simulink model "EsamblajeCohete2_0"  (R2023a)
settings: Solver=VariableStepAuto  StartTime=0.0  StopTime=120  RelTol=1e-3
model workspace: external: MATLAB File C:\Users\SEBASTIANDIAZPABON\OneDrive - Universidad Santo Tomás Bucaramanga\USTA\Semillero Cohete\Cohete Matlab 2.0\EsamblajeCohete2_0_DataFile.m (data not in the file)
undefined symbols (not defined in the file): smiData, X, Y, Z
libraries: sm_lib x354, nesl_utility x13, simulink x7, fuzblock x6
(part 7 of 7)

== system EsamblajeCohete2_0/Cohete/Assembly_4_RIGID/Magnet_8_RIGID ==
  ReferenceFrame : sm_lib/Frames and Transforms/Reference Frame
  Solid : sm_lib/Body Elements/File Solid  ExtGeomFileName=Magnet_Default_sldprt.STEP  UnitType=FromFile  ExtGeomFileUnits=m  StepReaderType=HEX  ExportConvexHullGeometry=off  InertiaType=Custom  Mass=smiData.Solid(5).mass  MassUnits=kg  CenterOfMass=smiData.Solid(5).CoM  CenterOfMassUnits=mm  MomentsOfInertia=smiData.Solid(5).MoI  MomentsOfInertiaUnits=kg*mm^2  ProductsOfInertia=smiData.Solid(5).PoI  ProductsOfInertiaUnits=kg*mm^2  BasedOnType=DensityFromFile  Density=1000  DensityUnits=kg/m^3  DoExposeReferenceFrame=on  SerializedFrames=<Frames/>  GraphicType=FromGeometry  MarkerShape=Sphere  MarkerSize=10  GraphicVisPropType=SimpleVisualProperties  GraphicDiffuseColor=smiData.Solid(5).color  GraphicSpecularColor=[0.5 0.5 0.5 1.0]  GraphicAmbientColor=[0.15 0.15 0.15 1.0]  GraphicEmissiveColor=[0.0 0.0 0.0 1.0]  GraphicShininess=75  GraphicOpacity=smiData.Solid(5).opacity
  F : PMIOPort  Side=Left
  connections:
  Solid/RConn1 -- ReferenceFrame/RConn1 -- F/RConn1

== system EsamblajeCohete2_0/Cohete/Assembly_4_RIGID/Magnet_9_RIGID ==
  ReferenceFrame : sm_lib/Frames and Transforms/Reference Frame
  Solid : sm_lib/Body Elements/File Solid  ExtGeomFileName=Magnet_Default_sldprt.STEP  UnitType=FromFile  ExtGeomFileUnits=m  StepReaderType=HEX  ExportConvexHullGeometry=off  InertiaType=Custom  Mass=smiData.Solid(5).mass  MassUnits=kg  CenterOfMass=smiData.Solid(5).CoM  CenterOfMassUnits=mm  MomentsOfInertia=smiData.Solid(5).MoI  MomentsOfInertiaUnits=kg*mm^2  ProductsOfInertia=smiData.Solid(5).PoI  ProductsOfInertiaUnits=kg*mm^2  BasedOnType=DensityFromFile  Density=1000  DensityUnits=kg/m^3  DoExposeReferenceFrame=on  SerializedFrames=<Frames/>  GraphicType=FromGeometry  MarkerShape=Sphere  MarkerSize=10  GraphicVisPropType=SimpleVisualProperties  GraphicDiffuseColor=smiData.Solid(5).color  GraphicSpecularColor=[0.5 0.5 0.5 1.0]  GraphicAmbientColor=[0.15 0.15 0.15 1.0]  GraphicEmissiveColor=[0.0 0.0 0.0 1.0]  GraphicShininess=75  GraphicOpacity=smiData.Solid(5).opacity
  F : PMIOPort  Side=Left
  connections:
  Solid/RConn1 -- ReferenceFrame/RConn1 -- F/RConn1

== system EsamblajeCohete2_0/Cohete/Assembly_4_RIGID/Motor_Casing_1_RIGID ==
  ReferenceFrame : sm_lib/Frames and Transforms/Reference Frame
  Solid : sm_lib/Body Elements/File Solid  ExtGeomFileName=Motor Casing_Default_sldprt.STEP  UnitType=FromFile  ExtGeomFileUnits=m  StepReaderType=HEX  ExportConvexHullGeometry=off  InertiaType=Custom  Mass=smiData.Solid(8).mass  MassUnits=kg  CenterOfMass=smiData.Solid(8).CoM  CenterOfMassUnits=mm  MomentsOfInertia=smiData.Solid(8).MoI  MomentsOfInertiaUnits=kg*mm^2  ProductsOfInertia=smiData.Solid(8).PoI  ProductsOfInertiaUnits=kg*mm^2  BasedOnType=DensityFromFile  Density=1000  DensityUnits=kg/m^3  DoExposeReferenceFrame=on  SerializedFrames=<Frames/>  GraphicType=FromGeometry  MarkerShape=Sphere  MarkerSize=10  GraphicVisPropType=SimpleVisualProperties  GraphicDiffuseColor=smiData.Solid(8).color  GraphicSpecularColor=[0.5 0.5 0.5 1.0]  GraphicAmbientColor=[0.15 0.15 0.15 1.0]  GraphicEmissiveColor=[0.0 0.0 0.0 1.0]  GraphicShininess=75  GraphicOpacity=smiData.Solid(8).opacity
  F : PMIOPort  Side=Left
  connections:
  Solid/RConn1 -- ReferenceFrame/RConn1 -- F/RConn1

== system EsamblajeCohete2_0/Cohete/Assembly_4_RIGID/Nut_2_RIGID ==
  ReferenceFrame : sm_lib/Frames and Transforms/Reference Frame
  Solid : sm_lib/Body Elements/File Solid  ExtGeomFileName=Nut_Default_sldprt.STEP  UnitType=FromFile  ExtGeomFileUnits=m  StepReaderType=HEX  ExportConvexHullGeometry=off  InertiaType=Custom  Mass=smiData.Solid(13).mass  MassUnits=kg  CenterOfMass=smiData.Solid(13).CoM  CenterOfMassUnits=mm  MomentsOfInertia=smiData.Solid(13).MoI  MomentsOfInertiaUnits=kg*mm^2  ProductsOfInertia=smiData.Solid(13).PoI  ProductsOfInertiaUnits=kg*mm^2  BasedOnType=DensityFromFile  Density=1000  DensityUnits=kg/m^3  DoExposeReferenceFrame=on  SerializedFrames=<Frames/>  GraphicType=FromGeometry  MarkerShape=Sphere  MarkerSize=10  GraphicVisPropType=SimpleVisualProperties  GraphicDiffuseColor=smiData.Solid(13).color  GraphicSpecularColor=[0.5 0.5 0.5 1.0]  GraphicAmbientColor=[0.15 0.15 0.15 1.0]  GraphicEmissiveColor=[0.0 0.0 0.0 1.0]  GraphicShininess=75  GraphicOpacity=smiData.Solid(13).opacity
  F : PMIOPort  Side=Left
  connections:
  Solid/RConn1 -- ReferenceFrame/RConn1 -- F/RConn1

== system EsamblajeCohete2_0/Cohete/Assembly_4_RIGID/Rotor_1_RIGID ==
  ReferenceFrame : sm_lib/Frames and Transforms/Reference Frame
  Solid : sm_lib/Body Elements/File Solid  ExtGeomFileName=Rotor_Default_sldprt.STEP  UnitType=FromFile  ExtGeomFileUnits=m  StepReaderType=HEX  ExportConvexHullGeometry=off  InertiaType=Custom  Mass=smiData.Solid(9).mass  MassUnits=kg  CenterOfMass=smiData.Solid(9).CoM  CenterOfMassUnits=mm  MomentsOfInertia=smiData.Solid(9).MoI  MomentsOfInertiaUnits=kg*mm^2  ProductsOfInertia=smiData.Solid(9).PoI  ProductsOfInertiaUnits=kg*mm^2  BasedOnType=DensityFromFile  Density=1000  DensityUnits=kg/m^3  DoExposeReferenceFrame=on  SerializedFrames=<Frames/>  GraphicType=FromGeometry  MarkerShape=Sphere  MarkerSize=10  GraphicVisPropType=SimpleVisualProperties  GraphicDiffuseColor=smiData.Solid(9).color  GraphicSpecularColor=[0.5 0.5 0.5 1.0]  GraphicAmbientColor=[0.15 0.15 0.15 1.0]  GraphicEmissiveColor=[0.0 0.0 0.0 1.0]  GraphicShininess=75  GraphicOpacity=smiData.Solid(9).opacity
  F : PMIOPort  Side=Left
  connections:
  Solid/RConn1 -- ReferenceFrame/RConn1 -- F/RConn1

== system EsamblajeCohete2_0/Cohete/Assembly_4_RIGID/Rotor_Cover_1_RIGID ==
  ReferenceFrame : sm_lib/Frames and Transforms/Reference Frame
  Solid : sm_lib/Body Elements/File Solid  ExtGeomFileName=Rotor Cover_Default_sldprt.STEP  UnitType=FromFile  ExtGeomFileUnits=m  StepReaderType=HEX  ExportConvexHullGeometry=off  InertiaType=Custom  Mass=smiData.Solid(11).mass  MassUnits=kg  CenterOfMass=smiData.Solid(11).CoM  CenterOfMassUnits=mm  MomentsOfInertia=smiData.Solid(11).MoI  MomentsOfInertiaUnits=kg*mm^2  ProductsOfInertia=smiData.Solid(11).PoI  ProductsOfInertiaUnits=kg*mm^2  BasedOnType=DensityFromFile  Density=1000  DensityUnits=kg/m^3  DoExposeReferenceFrame=on  SerializedFrames=<Frames/>  GraphicType=FromGeometry  MarkerShape=Sphere  MarkerSize=10  GraphicVisPropType=SimpleVisualProperties  GraphicDiffuseColor=smiData.Solid(11).color  GraphicSpecularColor=[0.5 0.5 0.5 1.0]  GraphicAmbientColor=[0.15 0.15 0.15 1.0]  GraphicEmissiveColor=[0.0 0.0 0.0 1.0]  GraphicShininess=75  GraphicOpacity=smiData.Solid(11).opacity
  F : PMIOPort  Side=Left
  connections:
  Solid/RConn1 -- ReferenceFrame/RConn1 -- F/RConn1

== system EsamblajeCohete2_0/Cohete/Assembly_4_RIGID/Stopper_Screw_1_RIGID ==
  ReferenceFrame : sm_lib/Frames and Transforms/Reference Frame
  Solid : sm_lib/Body Elements/File Solid  ExtGeomFileName=Stopper Screw_Default_sldprt.STEP  UnitType=FromFile  ExtGeomFileUnits=m  StepReaderType=HEX  ExportConvexHullGeometry=off  InertiaType=Custom  Mass=smiData.Solid(12).mass  MassUnits=kg  CenterOfMass=smiData.Solid(12).CoM  CenterOfMassUnits=mm  MomentsOfInertia=smiData.Solid(12).MoI  MomentsOfInertiaUnits=kg*mm^2  ProductsOfInertia=smiData.Solid(12).PoI  ProductsOfInertiaUnits=kg*mm^2  BasedOnType=DensityFromFile  Density=1000  DensityUnits=kg/m^3  DoExposeReferenceFrame=on  SerializedFrames=<Frames/>  GraphicType=FromGeometry  MarkerShape=Sphere  MarkerSize=10  GraphicVisPropType=SimpleVisualProperties  GraphicDiffuseColor=smiData.Solid(12).color  GraphicSpecularColor=[0.5 0.5 0.5 1.0]  GraphicAmbientColor=[0.15 0.15 0.15 1.0]  GraphicEmissiveColor=[0.0 0.0 0.0 1.0]  GraphicShininess=75  GraphicOpacity=smiData.Solid(12).opacity
  F : PMIOPort  Side=Left
  connections:
  Solid/RConn1 -- ReferenceFrame/RConn1 -- F/RConn1

== system EsamblajeCohete2_0/Cohete/Assembly_4_RIGID/e_ring_external_retaining_ring_wti_4_RIGID ==
  ReferenceFrame : sm_lib/Frames and Transforms/Reference Frame
  Solid : sm_lib/Body Elements/File Solid  ExtGeomFileName=e-ring external retaining ring_wti_Truarc X5133-14 - S0.14_sldprt.STEP  UnitType=FromFile  ExtGeomFileUnits=m  StepReaderType=HEX  ExportConvexHullGeometry=off  InertiaType=Custom  Mass=smiData.Solid(10).mass  MassUnits=kg  CenterOfMass=smiData.Solid(10).CoM  CenterOfMassUnits=in  MomentsOfInertia=smiData.Solid(10).MoI  MomentsOfInertiaUnits=kg*in^2  ProductsOfInertia=smiData.Solid(10).PoI  ProductsOfInertiaUnits=kg*in^2  BasedOnType=DensityFromFile  Density=1000  DensityUnits=kg/m^3  DoExposeReferenceFrame=on  SerializedFrames=<Frames/>  GraphicType=FromGeometry  MarkerShape=Sphere  MarkerSize=10  GraphicVisPropType=SimpleVisualProperties  GraphicDiffuseColor=smiData.Solid(10).color  GraphicSpecularColor=[0.5 0.5 0.5 1.0]  GraphicAmbientColor=[0.15 0.15 0.15 1.0]  GraphicEmissiveColor=[0.0 0.0 0.0 1.0]  GraphicShininess=75  GraphicOpacity=smiData.Solid(10).opacity
  F : PMIOPort  Side=Left
  connections:
  Solid/RConn1 -- ReferenceFrame/RConn1 -- F/RConn1

== system EsamblajeCohete2_0/Cohete/Assembly_4_RIGID/instrument_ball_bearing_68_iso_1_RIGID ==
  ReferenceFrame : sm_lib/Frames and Transforms/Reference Frame
  Solid : sm_lib/Body Elements/File Solid  ExtGeomFileName=instrument ball bearing_68_iso_ISO 1224 - 390308 - R-8-DE-NC-8_68_sldprt.STEP  UnitType=FromFile  ExtGeomFileUnits=m  StepReaderType=HEX  ExportConvexHullGeometry=off  InertiaType=Custom  Mass=smiData.Solid(14).mass  MassUnits=kg  CenterOfMass=smiData.Solid(14).CoM  CenterOfMassUnits=mm  MomentsOfInertia=smiData.Solid(14).MoI  MomentsOfInertiaUnits=kg*mm^2  ProductsOfInertia=smiData.Solid(14).PoI  ProductsOfInertiaUnits=kg*mm^2  BasedOnType=DensityFromFile  Density=1000  DensityUnits=kg/m^3  DoExposeReferenceFrame=on  SerializedFrames=<Frames/>  GraphicType=FromGeometry  MarkerShape=Sphere  MarkerSize=10  GraphicVisPropType=SimpleVisualProperties  GraphicDiffuseColor=smiData.Solid(14).color  GraphicSpecularColor=[0.5 0.5 0.5 1.0]  GraphicAmbientColor=[0.15 0.15 0.15 1.0]  GraphicEmissiveColor=[0.0 0.0 0.0 1.0]  GraphicShininess=75  GraphicOpacity=smiData.Solid(14).opacity
  F : PMIOPort  Side=Left
  connections:
  Solid/RConn1 -- ReferenceFrame/RConn1 -- F/RConn1

== system EsamblajeCohete2_0/Controlador + Planta/PID ADTITUDE/PID ATITUDE ==
  Z : Inport
  Z_error : Inport  Port=2
  Add : Sum  Inputs=+++
  Derivative : Derivative
  Integrator : Integrator
  Kda : Gain  Gain=1.5789
  Kia : Gain  Gain=0.021147
  Kpa : Gain  Gain=0.36
  Sum : Sum  Inputs=|+-
  Transfer Fcn : TransferFcn  Denominator=[1.6 0 0]
  z : Outport
  wires:
  Derivative/1 -> Add/3
  Integrator/1 -> Add/2
  Kpa/1 -> Add/1
  Sum/1 -> Kda/1, Kia/1, Kpa/1
  Z/1 -> Sum/1
  Z_error/1 -> Sum/2
  Kia/1 -> Integrator/1
  Kda/1 -> Derivative/1
  Add/1 -> Transfer Fcn/1
  Transfer Fcn/1 -> z/1

== system EsamblajeCohete2_0/Controlador + Planta/PID ADTITUDE/PID ATITUDE X ==
  X_d : Inport
  X_er : Inport  Port=2
  Add : Sum  Inputs=+++
  Add1 : Sum  Commented=on  Inputs=+-+-
  Derivative : Derivative
  Integrator : Integrator
  Kda : Gain  Gain=1.5789
  Kia : Gain  Gain=0.021147
  Kpa : Gain  Gain=0.36
  Ramp : simulink/Sources/Ramp  Commented=on  slope=0.1  start=18  InitialOutput=0
  Ramp1 : simulink/Sources/Ramp  Commented=on  slope=0.1  start=23  InitialOutput=0
  Step1 : Step  Commented=on  Time=24  After=0.12  SampleTime=0
  Step2 : Step  Commented=on  Time=24  After=0.62  SampleTime=0
  Sum : Sum  Inputs=|+-
  Sum1 : Sum  Inputs=|++
  Transfer Fcn : TransferFcn  Denominator=[1.6 0 0]
  z : Outport
  wires:
  Derivative/1 -> Add/3
  Integrator/1 -> Add/2
  Kpa/1 -> Add/1
  Sum/1 -> Kda/1, Kia/1, Kpa/1
  X_d/1 -> Sum/1
  X_er/1 -> Sum/2
  Kia/1 -> Integrator/1
  Kda/1 -> Derivative/1
  Add/1 -> Transfer Fcn/1
  Transfer Fcn/1 -> Sum1/1
  Sum1/1 -> z/1
  Ramp/1 -> Add1/1
  Ramp1/1 -> Add1/2
  Step1/1 -> Add1/3
  Step2/1 -> Add1/4
  Add1/1 -> Sum1/2

== system EsamblajeCohete2_0/Controlador + Planta/PID ADTITUDE/PID ATITUDE y  ==
  Z : Inport
  Z_error : Inport  Port=2
  Add : Sum  Inputs=+++
  Derivative : Derivative
  Integrator : Integrator
  Kda : Gain  Gain=1.5789
  Kia : Gain  Gain=0.021147
  Kpa : Gain  Gain=0.36
  Sum : Sum  Inputs=|+-
  Transfer Fcn : TransferFcn  Denominator=[1.6 0 0]
  z : Outport
  wires:
  Derivative/1 -> Add/3
  Integrator/1 -> Add/2
  Kpa/1 -> Add/1
  Sum/1 -> Kda/1, Kia/1, Kpa/1
  Z/1 -> Sum/1
  Z_error/1 -> Sum/2
  Kia/1 -> Integrator/1
  Kda/1 -> Derivative/1
  Add/1 -> Transfer Fcn/1
  Transfer Fcn/1 -> z/1

== system EsamblajeCohete2_0/Controlador + Planta/Rotation PID/PID θ ==
  θ : Inport
  θ_error : Inport  Port=2
  Add : Sum  Inputs=+++
  Derivative : Derivative
  Integrator : Integrator
  Kda : Gain  Gain=0.03947
  Kia : Gain  Gain=0.0005287
  Kpa : Gain  Gain=0.009136
  Sum : Sum  Inputs=|+-
  Transfer Fcn : TransferFcn  Denominator=[0.02 0 0]
  theta : Outport
  wires:
  Derivative/1 -> Add/3
  Integrator/1 -> Add/2
  Kpa/1 -> Add/1
  Sum/1 -> Kda/1, Kia/1, Kpa/1
  θ/1 -> Sum/1
  θ_error/1 -> Sum/2
  Kia/1 -> Integrator/1
  Kda/1 -> Derivative/1
  Add/1 -> Transfer Fcn/1
  Transfer Fcn/1 -> theta/1

== system EsamblajeCohete2_0/Controlador + Planta/Rotation PID/PID φ ==
  φ : Inport
  φ_error : Inport  Port=2
  Add : Sum  Inputs=+++
  Derivative : Derivative
  Integrator : Integrator
  Kda : Gain  Gain=0.01973
  Kia : Gain  Gain=0.00026434
  Kpa : Gain  Gain=0.0045681
  Sum : Sum  Inputs=|+-
  Transfer Fcn : TransferFcn  Denominator=[0.04 0 0]
  Out1 : Outport
  wires:
  Derivative/1 -> Add/3
  Integrator/1 -> Add/2
  Kpa/1 -> Add/1
  Sum/1 -> Kda/1, Kia/1, Kpa/1
  φ/1 -> Sum/1
  φ_error/1 -> Sum/2
  Kia/1 -> Integrator/1
  Kda/1 -> Derivative/1
  Add/1 -> Transfer Fcn/1
  Transfer Fcn/1 -> Out1/1

== system EsamblajeCohete2_0/Controlador + Planta/Rotation PID/PID ψ ==
  ψ : Inport
  ψ_error : Inport  Port=2
  Add : Sum  Inputs=+++
  Derivative : Derivative
  Integrator : Integrator
  Kda : Gain  Gain=0.03947
  Kia : Gain  Gain=0.0005287
  Kpa : Gain  Gain=0.009136
  Sum : Sum  Inputs=|+-
  Transfer Fcn : TransferFcn  Denominator=[0.02 0 0]
  theta : Outport
  wires:
  Derivative/1 -> Add/3
  Integrator/1 -> Add/2
  Kpa/1 -> Add/1
  Sum/1 -> Kda/1, Kia/1, Kpa/1
  ψ/1 -> Sum/1
  ψ_error/1 -> Sum/2
  Kia/1 -> Integrator/1
  Kda/1 -> Derivative/1
  Add/1 -> Transfer Fcn/1
  Transfer Fcn/1 -> theta/1

== system EsamblajeCohete2_0/Qudrotor Dinamics/Rotacional/θ'' ==
  Iyy : Inport
  Izz : Inport  Port=2
  Ixx : Inport  Port=3
  φ' : Inport  Port=4
  ψ' : Inport  Port=5
  L : Inport  Port=6
  U3 : Inport  Port=7
  Add : Sum  Inputs=+-
  Add1 : Sum
  Divide : Product  Inputs=*/
  Divide1 : Product  Inputs=*/
  Product : Product
  Product1 : Product  Inputs=3
  θ'' : Outport
  wires:
  Add/1 -> Divide/1
  Divide/1 -> Product1/1
  Product/1 -> Divide1/1
  Product1/1 -> Add1/1
  Divide1/1 -> Add1/2
  Add1/1 -> θ''/1
  Iyy/1 -> Divide1/2, Divide/2
  Izz/1 -> Add/1
  Ixx/1 -> Add/2
  φ'/1 -> Product1/2
  ψ'/1 -> Product1/3
  L/1 -> Product/1
  U3/1 -> Product/2

== system EsamblajeCohete2_0/Qudrotor Dinamics/Rotacional/φ'' ==
  Iyy : Inport
  Izz : Inport  Port=2
  Ixx : Inport  Port=3
  θ' : Inport  Port=4
  ψ' : Inport  Port=5
  L : Inport  Port=6
  U2 : Inport  Port=7
  Add : Sum  Inputs=+-
  Add1 : Sum
  Divide : Product  Inputs=*/
  Divide1 : Product  Inputs=*/
  Product : Product
  Product1 : Product  Inputs=3
  φ'' : Outport
  wires:
  Iyy/1 -> Add/1
  Izz/1 -> Add/2
  Add/1 -> Divide/1
  Ixx/1 -> Divide1/2, Divide/2
  Divide/1 -> Product1/1
  θ'/1 -> Product1/2
  ψ'/1 -> Product1/3
  L/1 -> Product/1
  U2/1 -> Product/2
  Product/1 -> Divide1/1
  Product1/1 -> Add1/1
  Divide1/1 -> Add1/2
  Add1/1 -> φ''/1

== system EsamblajeCohete2_0/Qudrotor Dinamics/Rotacional/ψ'' ==
  Iyy : Inport
  Izz : Inport  Port=2
  Ixx : Inport  Port=3
  φ' : Inport  Port=4
  θ' : Inport  Port=5
  L : Inport  Port=6
  U4 : Inport  Port=7
  Add : Sum  Inputs=+-
  Add1 : Sum
  Divide : Product  Inputs=*/
  Divide1 : Product  Inputs=*/
  Product : Product
  Product1 : Product  Inputs=3
  ψ'' : Outport
  wires:
  Add/1 -> Divide/1
  Divide/1 -> Product1/1
  Product/1 -> Divide1/1
  Product1/1 -> Add1/1
  Divide1/1 -> Add1/2
  Add1/1 -> ψ''/1
  Iyy/1 -> Add/2
  Ixx/1 -> Add/1
  Izz/1 -> Divide1/2, Divide/2
  φ'/1 -> Product1/2
  θ'/1 -> Product1/3
  L/1 -> Product/1
  U4/1 -> Product/2

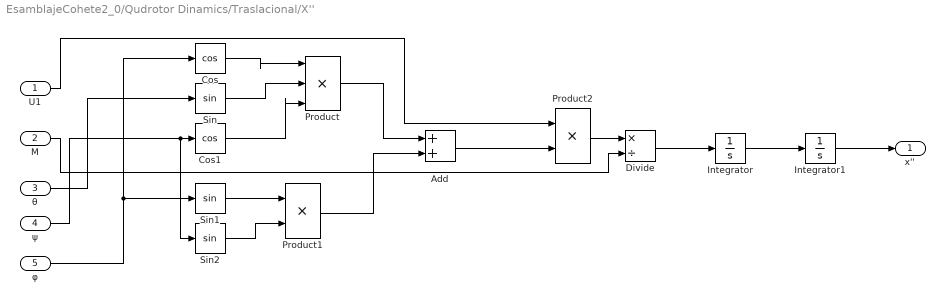
== system EsamblajeCohete2_0/Qudrotor Dinamics/Traslacional/X'' ==
  U1 : Inport
  M : Inport  Port=2
  θ : Inport  Port=3
  ψ : Inport  Port=4
  φ : Inport  Port=5
  Add : Sum
  Cos : Trigonometry  Operator=cos
  Cos1 : Trigonometry  Operator=cos
  Divide : Product  Inputs=*/
  Integrator : Integrator
  Integrator1 : Integrator
  Product : Product  Inputs=3
  Product1 : Product
  Product2 : Product
  Sin : Trigonometry
  Sin1 : Trigonometry
  Sin2 : Trigonometry
  x'' : Outport
  wires:
  φ/1 -> Sin1/1, Cos/1
  θ/1 -> Sin/1
  ψ/1 -> Sin2/1, Cos1/1
  Cos/1 -> Product/1
  Sin/1 -> Product/2
  Cos1/1 -> Product/3
  Product/1 -> Add/1
  Sin1/1 -> Product1/1
  Sin2/1 -> Product1/2
  Product1/1 -> Add/2
  U1/1 -> Product2/1
  Add/1 -> Product2/2
  Product2/1 -> Divide/1
  M/1 -> Divide/2
  Divide/1 -> Integrator/1
  Integrator/1 -> Integrator1/1
  Integrator1/1 -> x''/1

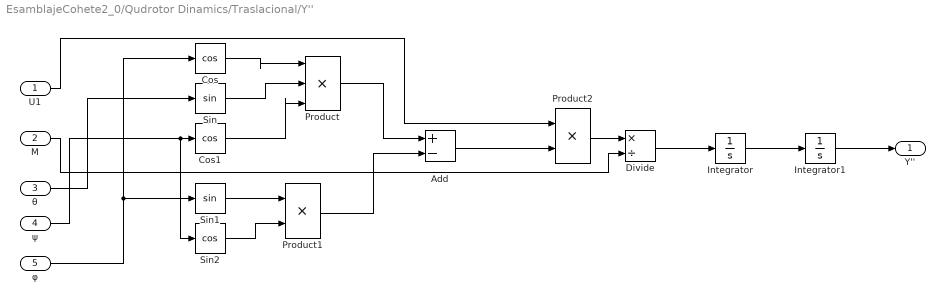
== system EsamblajeCohete2_0/Qudrotor Dinamics/Traslacional/Y'' ==
  U1 : Inport
  M : Inport  Port=2
  θ : Inport  Port=3
  ψ : Inport  Port=4
  φ : Inport  Port=5
  Add : Sum  Inputs=+-
  Cos : Trigonometry  Operator=cos
  Cos1 : Trigonometry  Operator=cos
  Divide : Product  Inputs=*/
  Integrator : Integrator
  Integrator1 : Integrator
  Product : Product  Inputs=3
  Product1 : Product
  Product2 : Product
  Sin : Trigonometry
  Sin1 : Trigonometry
  Sin2 : Trigonometry  Operator=cos
  Y'' : Outport
  wires:
  φ/1 -> Sin1/1, Cos/1
  θ/1 -> Sin/1
  ψ/1 -> Sin2/1, Cos1/1
  Cos/1 -> Product/1
  Sin/1 -> Product/2
  Cos1/1 -> Product/3
  Product/1 -> Add/1
  Sin1/1 -> Product1/1
  Sin2/1 -> Product1/2
  Product1/1 -> Add/2
  U1/1 -> Product2/1
  Add/1 -> Product2/2
  Product2/1 -> Divide/1
  M/1 -> Divide/2
  Divide/1 -> Integrator/1
  Integrator/1 -> Integrator1/1
  Integrator1/1 -> Y''/1

== system EsamblajeCohete2_0/Qudrotor Dinamics/Traslacional/Z'' ==
  g : Inport
  U1 : Inport  Port=2
  M : Inport  Port=3
  θ : Inport  Port=4
  ψ : Inport  Port=5
  Add : Sum  Inputs=-+
  Cosine : simulink/Lookup Tables/Cosine  Formula=cos(2*pi*u)  NumDataPoints=(2^5)+1  OutputWordLength=16  InternalRulePriority=Speed
  Cosine1 : simulink/Lookup Tables/Cosine  Formula=cos(2*pi*u)  NumDataPoints=(2^5)+1  OutputWordLength=16  InternalRulePriority=Speed
  Divide : Product  Inputs=*/
  Product : Product  Inputs=3
  Out1 : Outport
  wires:
  ψ/1 -> Cosine1/1
  U1/1 -> Product/1
  Add/1 -> Out1/1
  Cosine/1 -> Product/2
  Cosine1/1 -> Product/3
  M/1 -> Divide/2
  g/1 -> Add/1
  θ/1 -> Cosine/1
  Divide/1 -> Add/2
  Product/1 -> Divide/1
